simulink model "modelNew"  (R2015a)
settings: Solver=ode45  StartTime=0.0  StopTime=tsim  RelTol=1e-3
undefined symbols (not defined in the file): Aref, B, Bref, Ch, gamma, GammaR, GammaX, Kh, L, M, P, R
settings Model: Creator=user  LastModifiedBy=user

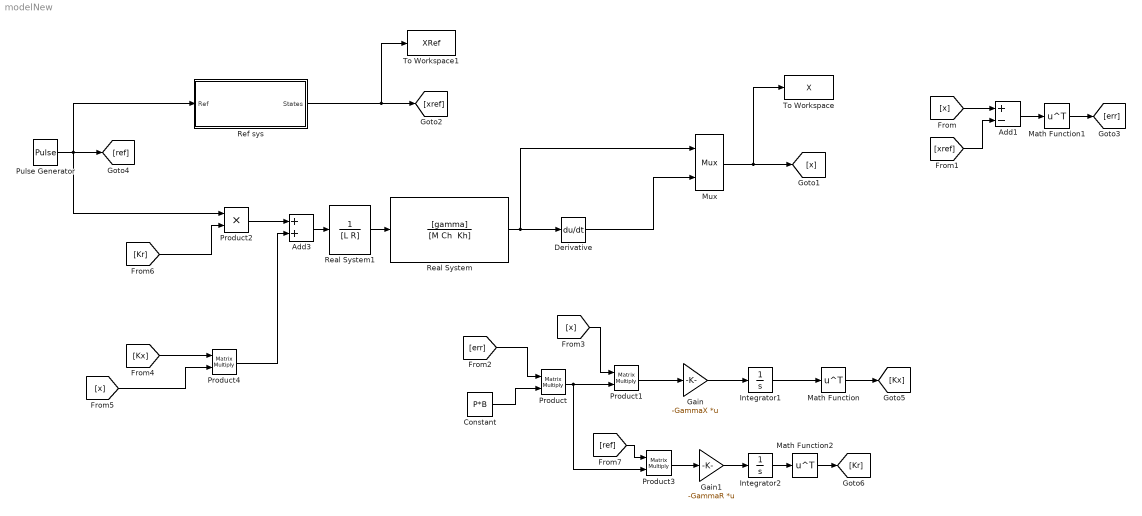
== system modelNew ==
  Add1 : Sum  Inputs=+-
  Add3 : Sum
  Constant : Constant  Value=P*B
  Derivative : Derivative
  Gain : Gain  Gain=-GammaX  Multiplication=Matrix(K*u)
  Gain1 : Gain  Gain=-GammaR  Multiplication=Matrix(K*u)
  Integrator1 : Integrator
  Integrator2 : Integrator
  Math Function : Math  Operator=transpose  SaturateOnIntegerOverflow=on
  Math Function1 : Math  Operator=transpose  SaturateOnIntegerOverflow=on
  Math Function2 : Math  Operator=transpose  SaturateOnIntegerOverflow=on
  Mux : Mux  Inputs=2
  Product{,1,3..4} (4 alike) : Product  Multiplication=Matrix(*)
  Product2 : Product
  Pulse Generator : DiscretePulseGenerator  PulseType=Time based  Period=10  PulseWidth=50
  Real System : TransferFcn  Numerator=[gamma]  Denominator="[M Ch  Kh]"
  Real System1 : TransferFcn  Numerator=1  Denominator=[L R]
  Ref sys : Subsystem
  To Workspace : ToWorkspace  VariableName=X  SaveFormat=Timeseries  SampleTime=1/200
  To Workspace1 : ToWorkspace  VariableName=XRef  SaveFormat=Timeseries  SampleTime=1/200
  wires:
  Pulse Generator/1 -> [ref], Product2/1, Ref sys/1(Ref)
  Ref sys/1(States) -> To Workspace1/1, [xref]
  Real System/1 -> Mux/1, Derivative/1
  Derivative/1 -> Mux/2
  [x] -> Add1/1
  [xref] -> Add1/2
  [err] -> Product/1
  Constant/1 -> Product/2
  Product/1 -> Product3/2, Product1/2
  [x] -> Product1/1
  Product1/1 -> Gain/1
  Gain/1 -> Integrator1/1
  Integrator1/1 -> Math Function/1
  Add1/1 -> Math Function1/1
  Math Function1/1 -> [err]
  [Kr] -> Product2/2
  Product2/1 -> Add3/1
  Product4/1 -> Add3/2
  Real System1/1 -> Real System/1
  Add3/1 -> Real System1/1
  Mux/1 -> To Workspace/1, [x]
  [Kx] -> Product4/1
  [x] -> Product4/2
  [ref] -> Product3/1
  Product3/1 -> Gain1/1
  Gain1/1 -> Integrator2/1
  Integrator2/1 -> Math Function2/1
  Math Function/1 -> [Kx]
  Math Function2/1 -> [Kr]

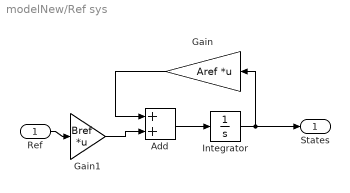
== system modelNew/Ref sys ==
  Ref : Inport
  Add : Sum
  Gain : Gain  Gain=Aref  Multiplication=Matrix(K*u)
  Gain1 : Gain  Gain=Bref  Multiplication=Matrix(K*u)
  Integrator : Integrator
  States : Outport
  wires:
  Gain/1 -> Add/1
  Gain1/1 -> Add/2
  Add/1 -> Integrator/1
  Ref/1 -> Gain1/1
  Integrator/1 -> States/1, Gain/1
